simulink library "TurtleCtrlLib"  (R2017a)
settings: Solver=VariableStepAuto  StartTime=0.0  StopTime=10.0  RelTol=1e-3
undefined symbols (not defined in the file or in its folder): Angular, Linear, magnitude
libraries: simulink x7, robotlib x2
settings Model: Creator=igeorgie  LastModifiedBy=igeorgie

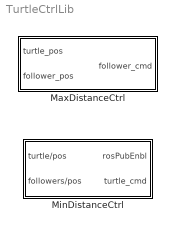
== system TurtleCtrlLib ==
  MaxDistanceCtrl : Subsystem  mask{p_gain_linear=1, p_gain_angular=10, max_distance=3}
  MinDistanceCtrl : Subsystem

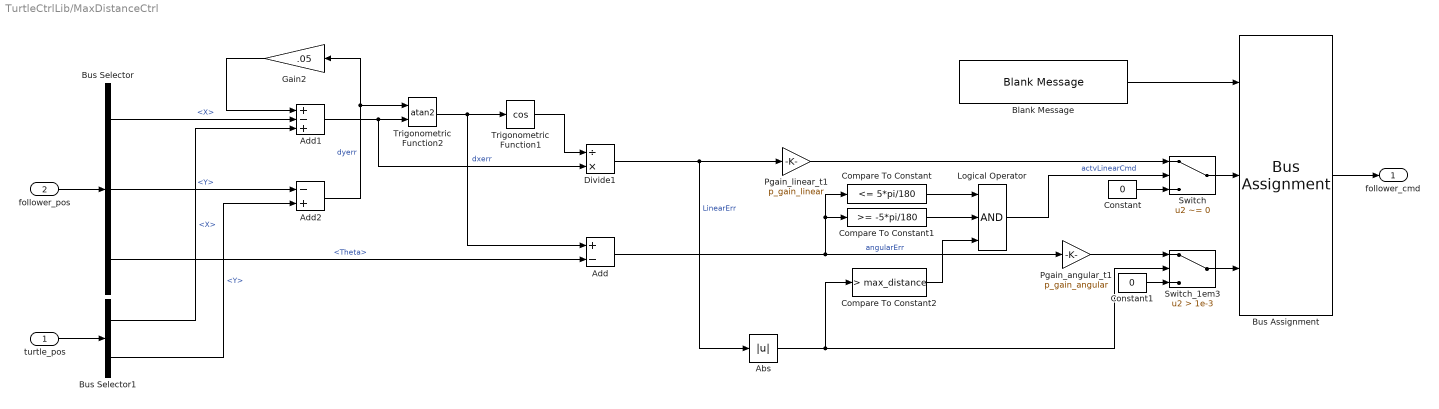
== system TurtleCtrlLib/MaxDistanceCtrl ==
  turtle_pos : Inport
  follower_pos : Inport  Port=2
  Abs : Abs
  Add : Sum  Inputs=+-
  Add1 : Sum  Inputs=+-+
  Add2 : Sum  Inputs=-+
  Blank Message : robotlib/Blank Message  SourceLibraryInfo=This block requires Robotics System Toolbox  messageType=geometry_msgs/Twist  SampleTime=inf
      settings: SourceProductBaseCode=RO
  Bus Assignment : BusAssignment  AssignedSignals=Linear.X,Angular.Z
  Bus Selector : BusSelector  OutputSignals=X,Y,Theta
  Bus Selector1 : BusSelector  OutputSignals=X,Y
  Compare To Constant : simulink/Logic and Bit Operations/Compare To Constant  relop=<=  const=5*pi/180  OutDataTypeStr=boolean
  Compare To Constant1 : simulink/Logic and Bit Operations/Compare To Constant  relop=>=  const=-5*pi/180  OutDataTypeStr=boolean
  Compare To Constant2 : simulink/Logic and Bit Operations/Compare To Constant  relop=>  const=max_distance  OutDataTypeStr=boolean
  Constant : Constant  Value=0
  Constant1 : Constant  Value=0
  Divide1 : Product  Inputs=/*
  Gain2 : Gain  Gain=.05
  Logical Operator : Logic  Inputs=3  AllPortsSameDT=off  OutDataTypeStr=boolean
  Pgain_angular_t1 : Gain  Gain=p_gain_angular
  Pgain_linear_t1 : Gain  Gain=p_gain_linear
  Switch : Switch  Criteria=u2 ~= 0
  Switch_1em3 : Switch  Criteria=u2 > Threshold  Threshold=1e-3
  Trigonometric Function1 : Trigonometry  Operator=cos
  Trigonometric Function2 : Trigonometry  Operator=atan2
  follower_cmd : Outport
  wires:
  Bus Selector1/2 -> Add2/2  "<Y>"
  Bus Selector1/1 -> Add1/3  "<X>"
  Constant1/1 -> Switch_1em3/3
  Abs/1 -> Switch_1em3/2, Compare To Constant2/1
  Switch_1em3/1 -> Bus Assignment/3
  Gain2/1 -> Add1/1
  Add/1 -> Compare To Constant/1, Compare To Constant1/1, Pgain_angular_t1/1  "angularErr"
  Bus Selector/3 -> Add/2  "<Theta>"
  Bus Selector/2 -> Add2/1  "<Y>"
  Bus Selector/1 -> Add1/2  "<X>"
  Bus Assignment/1 -> follower_cmd/1
  Blank Message/1 -> Bus Assignment/1
  Trigonometric Function2/1 -> Trigonometric Function1/1, Add/1
  Trigonometric Function1/1 -> Divide1/1
  Compare To Constant/1 -> Logical Operator/1
  Constant/1 -> Switch/3
  Divide1/1 -> Pgain_linear_t1/1, Abs/1  "LinearErr"
  Logical Operator/1 -> Switch/2  "actvLinearCmd"
  Add1/1 -> Divide1/2, Trigonometric Function2/2  "dxerr"
  Add2/1 -> Gain2/1, Trigonometric Function2/1  "dyerr"
  Switch/1 -> Bus Assignment/2
  Compare To Constant1/1 -> Logical Operator/2
  Pgain_linear_t1/1 -> Switch/1
  turtle_pos/1 -> Bus Selector1/1
  follower_pos/1 -> Bus Selector/1
  Compare To Constant2/1 -> Logical Operator/3
  Pgain_angular_t1/1 -> Switch_1em3/1

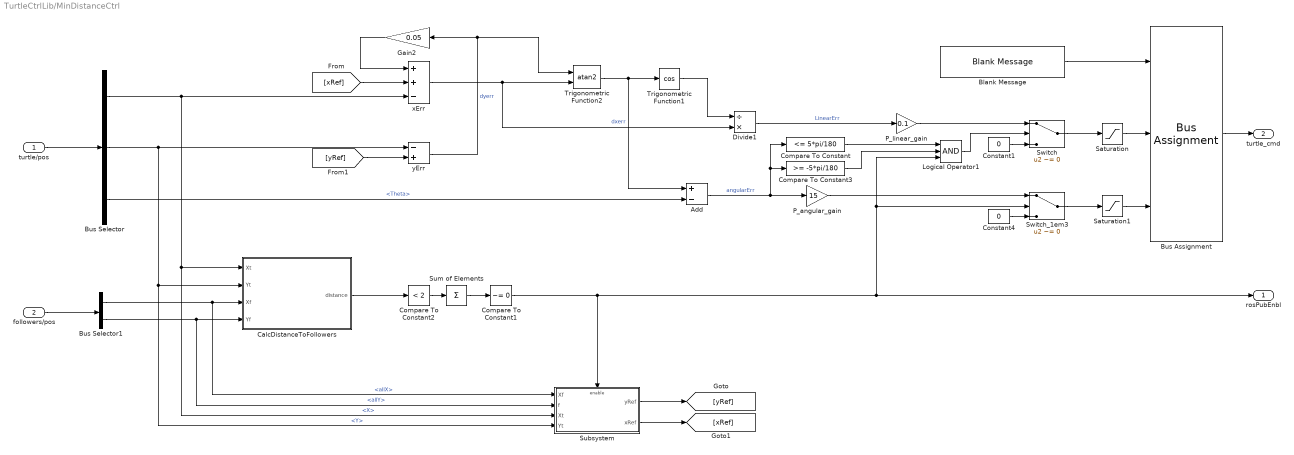
== system TurtleCtrlLib/MinDistanceCtrl ==
  turtle/pos : Inport
  followers/pos : Inport  Port=2
  Add : Sum  Inputs=+-
  Blank Message : robotlib/Blank Message  SourceLibraryInfo=This block requires Robotics System Toolbox  messageType=geometry_msgs/Twist  SampleTime=inf
      settings: SourceProductBaseCode=RO
  Bus Assignment : BusAssignment  AssignedSignals=Linear.X,Angular.Z
  Bus Selector : BusSelector  OutputSignals=X,Y,Theta
  Bus Selector1 : BusSelector  OutputSignals=allX,allY
  CalcDistanceToFollowers : Subsystem  TreatAsAtomicUnit=on
  Compare To Constant : simulink/Logic and Bit Operations/Compare To Constant  relop=<=  const=5*pi/180  OutDataTypeStr=boolean
  Compare To Constant1 : simulink/Logic and Bit Operations/Compare To Constant  relop=~=  const=0  OutDataTypeStr=boolean
  Compare To Constant2 : simulink/Logic and Bit Operations/Compare To Constant  relop=<  const=2  OutDataTypeStr=boolean
  Compare To Constant3 : simulink/Logic and Bit Operations/Compare To Constant  relop=>=  const=-5*pi/180  OutDataTypeStr=boolean
  Constant1 : Constant  Value=0
  Constant4 : Constant  Value=0
  Divide1 : Product  Inputs=/*
  Gain2 : Gain  Gain=0.05
  Logical Operator1 : Logic  Inputs=3  AllPortsSameDT=off  OutDataTypeStr=boolean
  P_angular_gain : Gain  Gain=15
  P_linear_gain : Gain  Gain=0.1
  Saturation : Saturate  UpperLimit=10  LowerLimit=-10
  Saturation1 : Saturate  UpperLimit=10  LowerLimit=-10
  Subsystem : Subsystem
  Sum of Elements : Sum  Inputs=+
  Switch : Switch  Criteria=u2 ~= 0
  Switch_1em3 : Switch  Criteria=u2 ~= 0  Threshold=1e-3
  Trigonometric Function1 : Trigonometry  Operator=cos
  Trigonometric Function2 : Trigonometry  Operator=atan2
  xErr : Sum  Inputs=++-
  yErr : Sum  Inputs=-+
  rosPubEnbl : Outport
  turtle_cmd : Outport  Port=2
  wires:
  Switch/1 -> Saturation/1
  P_angular_gain/1 -> Switch_1em3/1
  yErr/1 -> Trigonometric Function2/1, Gain2/1  "dyerr"
  xErr/1 -> Divide1/2, Trigonometric Function2/2  "dxerr"
  Divide1/1 -> P_linear_gain/1  "LinearErr"
  Trigonometric Function1/1 -> Divide1/1
  Trigonometric Function2/1 -> Add/1, Trigonometric Function1/1
  turtle/pos/1 -> Bus Selector/1
  Blank Message/1 -> Bus Assignment/1
  Bus Assignment/1 -> turtle_cmd/1
  Bus Selector/1 -> xErr/3, CalcDistanceToFollowers/1(Xt), Subsystem/3(Xt)  "<X>"
  Bus Selector/2 -> yErr/1, CalcDistanceToFollowers/2(Yt), Subsystem/4(Yt)  "<Y>"
  Bus Selector/3 -> Add/2  "<Theta>"
  Gain2/1 -> xErr/1
  Switch_1em3/1 -> Saturation1/1
  Sum of Elements/1 -> Compare To Constant1/1
  CalcDistanceToFollowers/1(distance) -> Compare To Constant2/1
  Compare To Constant2/1 -> Sum of Elements/1
  P_linear_gain/1 -> Switch/1
  Compare To Constant/1 -> Logical Operator1/1
  Compare To Constant3/1 -> Logical Operator1/2
  Add/1 -> Compare To Constant/1, Compare To Constant3/1, P_angular_gain/1  "angularErr"
  Logical Operator1/1 -> Switch/2
  Constant1/1 -> Switch/3
  Constant4/1 -> Switch_1em3/3
  Compare To Constant1/1 -> Switch_1em3/2, Logical Operator1/3, rosPubEnbl/1, Subsystem/Enable
  followers/pos/1 -> Bus Selector1/1
  Bus Selector1/1 -> Subsystem/1(Xf), CalcDistanceToFollowers/3(Xf)  "<allX>"
  Bus Selector1/2 -> Subsystem/2(f), CalcDistanceToFollowers/4(Yf)  "<allY>"
  [xRef] -> xErr/2
  [yRef] -> yErr/2
  Subsystem/1(yRef) -> [yRef]
  Subsystem/2(xRef) -> [xRef]
  Saturation/1 -> Bus Assignment/2
  Saturation1/1 -> Bus Assignment/3

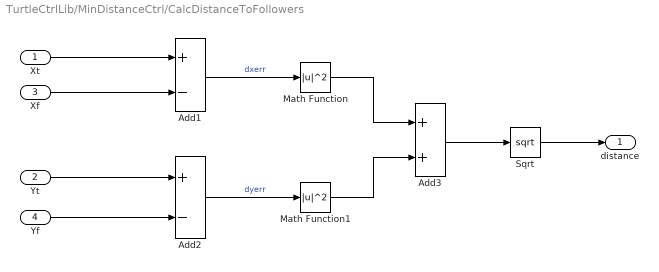
== system TurtleCtrlLib/MinDistanceCtrl/CalcDistanceToFollowers ==
  Xt : Inport
  Yt : Inport  Port=2
  Xf : Inport  Port=3
  Yf : Inport  Port=4
  Add1 : Sum  Inputs=+-
  Add2 : Sum  Inputs=+-
  Add3 : Sum
  Math Function : Math  Operator=magnitude^2  SaturateOnIntegerOverflow=on
  Math Function1 : Math  Operator=magnitude^2  SaturateOnIntegerOverflow=on
  Sqrt : Sqrt  SaturateOnIntegerOverflow=on
  distance : Outport
  wires:
  Yt/1 -> Add2/1
  Xf/1 -> Add1/2
  Math Function1/1 -> Add3/2
  Add2/1 -> Math Function1/1  "dyerr"
  Add3/1 -> Sqrt/1
  Yf/1 -> Add2/2
  Sqrt/1 -> distance/1
  Xt/1 -> Add1/1
  Add1/1 -> Math Function/1  "dxerr"
  Math Function/1 -> Add3/1

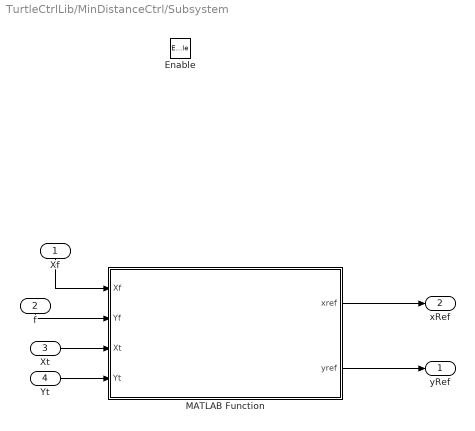
== system TurtleCtrlLib/MinDistanceCtrl/Subsystem ==
  Xf : Inport
  f : Inport  Port=2
  Xt : Inport  Port=3
  Yt : Inport  Port=4
  Enable : EnablePort
  MATLAB Function : MATLAB Function  TreatAsAtomicUnit=on
  yRef : Outport
  xRef : Outport  Port=2
  wires:
  f/1 -> MATLAB Function/2(Yf)
  Xf/1 -> MATLAB Function/1(Xf)
  Xt/1 -> MATLAB Function/3(Xt)
  Yt/1 -> MATLAB Function/4(Yt)
  MATLAB Function/1(xref) -> xRef/1
  MATLAB Function/2(yref) -> yRef/1

== matlab function TurtleCtrlLib/MinDistanceCtrl/Subsystem/MATLAB Function ==
  data: Xf input; xref output; Yf input; yref output; Xt input; Yt input
function [xref,yref]= fcn(Xf,Yf,Xt,Yt)

coeff_f = polyfit(Xf,Yf,1);

mean_xf = mean(Xf);
mean_yf = polyval(coeff_f,mean_xf)

fi=atan(coeff_f(1));
tan_fi=tan(fi);

if(tan_fi>0)
    si=(pi/2)+double(fi);
elseif(tan_fi<0)
    si=double(fi)-(pi/2);
else
    si=pi/2;
end

tan_si= tan(si)
b = mean_yf - mean_xf*tan_si;
coeff_t=[tan_si b];

y_tmp = polyval(coeff_f,Xt);
if(Yt > y_tmp && tan_fi>0) || (Yt < y_tmp && tan_fi<0)
    xref = double(mean_xf-3);
elseif(Yt > y_tmp && tan_fi<0) || (Yt < y_tmp && tan_fi>0)
    xref = double(mean_xf+3);
else
    xref=0;
end
yref = double(polyval(coeff_t,xref));
    
x = 0:0.1:10;
y1 = polyval(coeff_f,x);
y2 = polyval([tan_si b],x);

plot(x,y1,'--b',x,y2,'--g',Xf(1),Yf(1),'o',Xf(2),Yf(2),'o',Xf(3),Yf(3),'o',Xf(4),Yf(4),'o',xref,yref,'+',Xt,Yt,'^',mean_xf,mean_yf,'mx')
